simulink model "first_proto"  (R2023a)
settings: Solver=VariableStepAuto  StartTime=0.0  StopTime=10.0  RelTol=1e-3
settings Model: Creator=Алексей  LastModifiedBy=Алексей

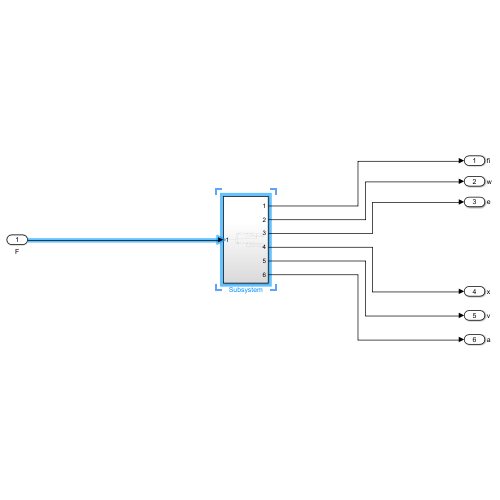
[thumbnail: Simulink's stored preview of the top-level diagram]
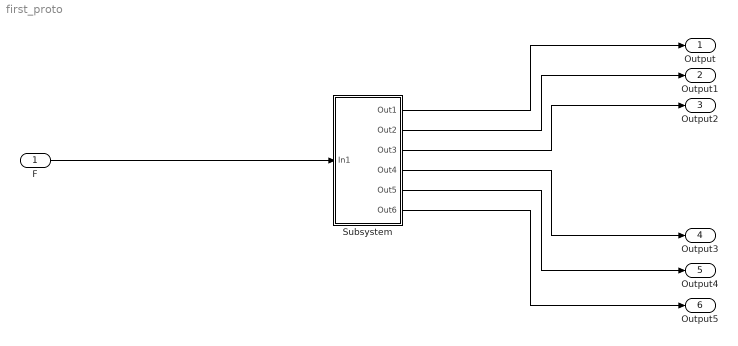
== system first_proto ==
  F : Inport
  Subsystem : Subsystem
  Output : Outport  SignalName=fi
  Output1 : Outport  Port=2  SignalName=w
  Output2 : Outport  Port=3  SignalName=e
  Output3 : Outport  Port=4  SignalName=x
  Output4 : Outport  Port=5  SignalName=v
  Output5 : Outport  Port=6  SignalName=a
  wires:
  F/1 -> Subsystem/1(In1)
  Subsystem/1(Out1) -> Output/1
  Subsystem/2(Out2) -> Output1/1
  Subsystem/3(Out3) -> Output2/1
  Subsystem/4(Out4) -> Output3/1
  Subsystem/5(Out5) -> Output4/1
  Subsystem/6(Out6) -> Output5/1

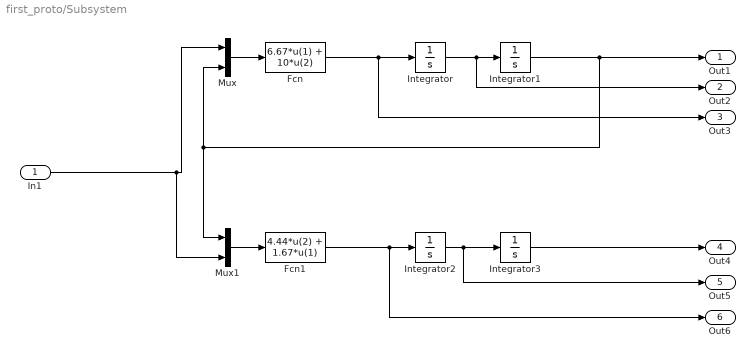
== system first_proto/Subsystem ==
  In1 : Inport
  Fcn : Fcn  Expr=6.67*u(1) + 10*u(2)
  Fcn1 : Fcn  Expr=4.44*u(2) + 1.67*u(1)
  Integrator : Integrator
  Integrator1 : Integrator  InitialCondition=5
  Integrator2 : Integrator
  Integrator3 : Integrator
  Mux : Mux  Inputs=2
  Mux1 : Mux  Inputs=2
  Out1 : Outport
  Out2 : Outport  Port=2
  Out3 : Outport  Port=3
  Out4 : Outport  Port=4
  Out5 : Outport  Port=5
  Out6 : Outport  Port=6
  wires:
  Mux/1 -> Fcn/1
  Integrator/1 -> Out2/1, Integrator1/1
  Fcn1/1 -> Out6/1, Integrator2/1
  Integrator3/1 -> Out4/1
  In1/1 -> Mux/1, Mux1/2
  Fcn/1 -> Out3/1, Integrator/1
  Integrator2/1 -> Out5/1, Integrator3/1
  Integrator1/1 -> Out1/1, Mux1/1, Mux/2
  Mux1/1 -> Fcn1/1
